simulink model "car4"  (R2016a)
settings: Solver=VariableStepAuto  StartTime=0.0  StopTime=20  RelTol=1e-3
libraries: simulink x1
settings Model: Creator=richa  LastModifiedBy=108

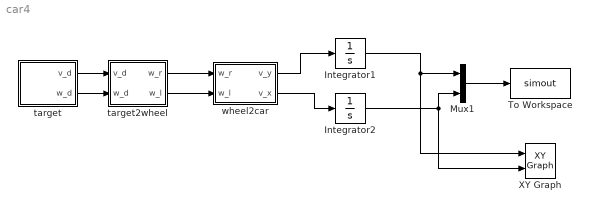
== system car4 ==
  Integrator1 : Integrator
  Integrator2 : Integrator
  Mux1 : Mux  Inputs=2
  To Workspace : ToWorkspace  VariableName=simout  SampleTime=-1
  XY Graph : simulink/Sinks/XY Graph  xmin=-2  xmax=2  ymin=-2  ymax=2  st=0
  target : Subsystem
  target2wheel : Subsystem
  wheel2car : Subsystem
  wires:
  Integrator1/1 -> Mux1/1, XY Graph/1
  Integrator2/1 -> Mux1/2, XY Graph/2
  Mux1/1 -> To Workspace/1
  wheel2car/1(v_y) -> Integrator1/1
  wheel2car/2(v_x) -> Integrator2/1
  target/2(w_d) -> target2wheel/2(w_d)
  target2wheel/1(w_r) -> wheel2car/1(w_r)
  target2wheel/2(w_l) -> wheel2car/2(w_l)
  target/1(v_d) -> target2wheel/1(v_d)

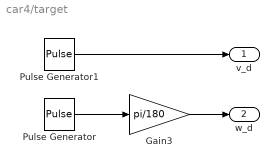
== system car4/target ==
  Gain3 : Gain  Gain=pi/180
  Pulse Generator : DiscretePulseGenerator  PulseType=Time based  Amplitude=90  PulseWidth=50  PhaseDelay=1
  Pulse Generator1 : DiscretePulseGenerator  PulseType=Time based  PulseWidth=50
  v_d : Outport
  w_d : Outport  Port=2
  wires:
  Pulse Generator/1 -> Gain3/1
  Pulse Generator1/1 -> v_d/1
  Gain3/1 -> w_d/1

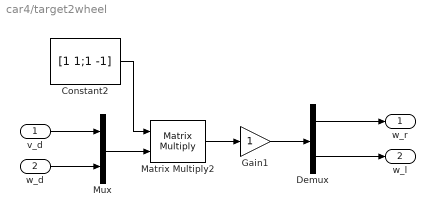
== system car4/target2wheel ==
  v_d : Inport
  w_d : Inport  Port=2
  Constant2 : Constant  Value=[1 1;1 -1]
  Demux : Demux  Outputs=2
  Gain1 : Gain
  Matrix Multiply2 : Product  Multiplication=Matrix(*)
  Mux : Mux  Inputs=2
  w_r : Outport
  w_l : Outport  Port=2
  wires:
  Mux/1 -> Matrix Multiply2/2
  Gain1/1 -> Demux/1
  Constant2/1 -> Matrix Multiply2/1
  Matrix Multiply2/1 -> Gain1/1
  v_d/1 -> Mux/1
  w_d/1 -> Mux/2
  Demux/2 -> w_l/1
  Demux/1 -> w_r/1

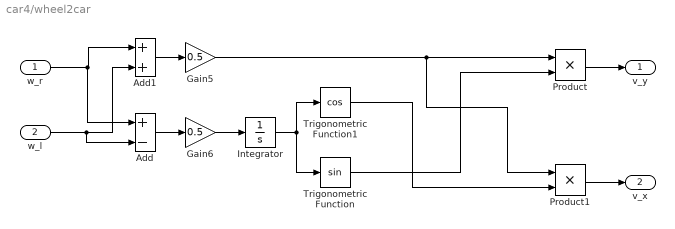
== system car4/wheel2car ==
  w_r : Inport
  w_l : Inport  Port=2
  Add : Sum  Inputs=+-
  Add1 : Sum
  Gain5 : Gain  Gain=0.5
  Gain6 : Gain  Gain=0.5
  Integrator : Integrator
  Product : Product
  Product1 : Product
  Trigonometric Function : Trigonometry
  Trigonometric Function1 : Trigonometry  Operator=cos
  v_y : Outport
  v_x : Outport  Port=2
  wires:
  Gain5/1 -> Product1/1, Product/1
  Gain6/1 -> Integrator/1
  Integrator/1 -> Trigonometric Function1/1, Trigonometric Function/1
  Trigonometric Function/1 -> Product/2
  Trigonometric Function1/1 -> Product1/2
  Product/1 -> v_y/1
  w_r/1 -> Add/1, Add1/1
  w_l/1 -> Add/2, Add1/2
  Product1/1 -> v_x/1
  Add1/1 -> Gain5/1
  Add/1 -> Gain6/1
